simulink model "doubleCond_tcarre"  (R2016b)
settings: Solver=VariableStepAuto  StartTime=0.0  StopTime=2  RelTol=1e-3
libraries: simulink x1
settings Model: Creator=live  LastModifiedBy=live

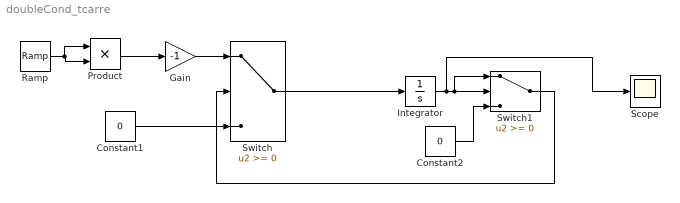
== system doubleCond_tcarre ==
  Constant1 : Constant  Value=0
  Constant2 : Constant  Value=0
  Gain : Gain  Gain=-1
  Integrator : Integrator  InitialCondition=1
  Product : Product
  Ramp : simulink/Sources/Ramp  slope=1  start=0  X0=0
  Scope : Scope
  Switch : Switch
  Switch1 : Switch
  wires:
  Constant1/1 -> Switch/3
  Switch/1 -> Integrator/1
  Integrator/1 -> Scope/1, Switch1/1, Switch1/2
  Constant2/1 -> Switch1/3
  Switch1/1 -> Switch/2
  Ramp/1 -> Product/1, Product/2
  Gain/1 -> Switch/1
  Product/1 -> Gain/1
